simulink model "gm_DUC_1"  (R2024b)
settings: Solver=FixedStepDiscrete  StartTime=0.0  StopTime=50000/fs_duc  FixedStep=1.62760416666667e-07  RelTol=1e-3
undefined symbols (not defined in the file or in its folder): compFilt, hbFilt, lowpassFilt
libraries: simulink x4, dsphdlfiltering2 x3, dsphdlsigops2 x2, hdlmdlgenlib x1, dspsigops x1
settings Model: Creator=31651  LastModifiedBy=31651
settings OptimizationCC: BlockReduction=off  ConditionallyExecuteInputs=off
settings DebuggingCC: SignalRangeChecking=warning  InheritedTsInSrcMsg=none  SingleTaskRateTransMsg=error  ParamPrecisionLossAbsoluteDiffThreshold=0.0001  ParamPrecisionLossRelativeDiffThreshold=0.0001
settings RTWCC: GPUComputeCapability=3.5

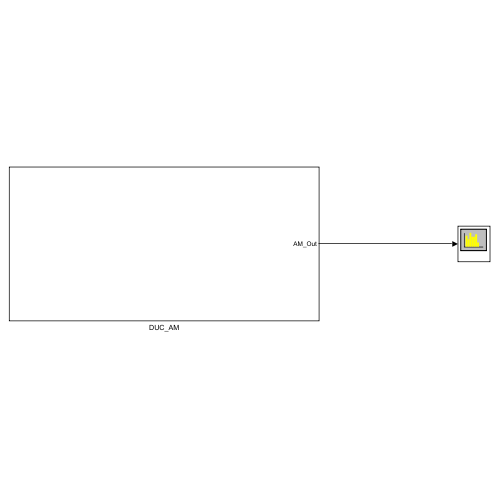
[thumbnail: Simulink's stored preview of the top-level diagram]
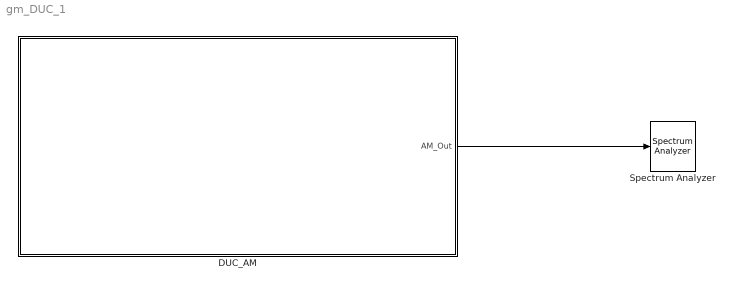
== system gm_DUC_1 ==
  DUC_AM : Subsystem
  Spectrum Analyzer : SpectrumAnalyzer  WindowPosition=[229.000000,148.000000,800.000000,500.000000,]  Visible=on  ScopeFrameLocation=window  SpectrumType=RMS  Method=Welch  WindowInvariantSamplesPerUpdate=on  Span=6144000  StartFrequency=-3072000  StopFrequency=3072000  SpectrumUnits=Vrms  YLimits=[-17.4955218,157.46114017]  SelectedToolstripTab=spectrumAnalyzerToolstrip.estimationTab
  wires:
  DUC_AM/1(AM_Out) -> Spectrum Analyzer/1

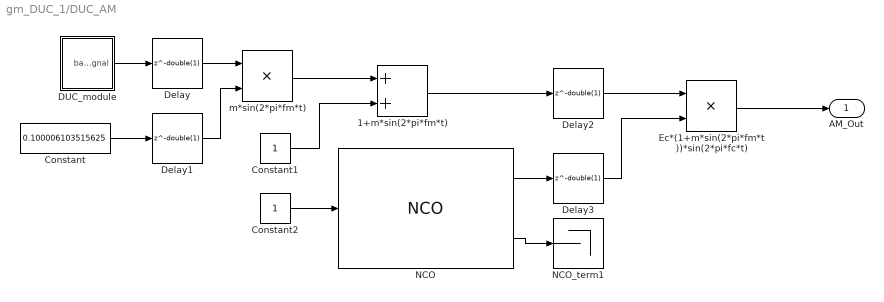
== system gm_DUC_1/DUC_AM ==
  1+m*sin(2*pi*fm*t) : Sum  OutDataTypeStr=fixdt(1, 32, 17)  AccumDataTypeStr=fixdt(1, 32, 17)  SampleTime=1.62760416666667e-07
  Constant : Constant  Value=0.100006103515625  OutDataTypeStr=fixdt(1, 16, 15)  SampleTime=1.62760416666667e-07
  Constant1 : Constant  OutDataTypeStr=int8  SampleTime=1.62760416666667e-07
  Constant2 : Constant  OutDataTypeStr=boolean  SampleTime=1.62760416666667e-07
  DUC_module : Subsystem
  Delay{,1..3} (4 alike) : Delay  DelayLength=double(1)  InitialCondition=0  SampleTime=1.62760416666667e-07
  Ec*(1+m*sin(2*pi*fm*t))*sin(2*pi*fc*t) : Product  Inputs=**  OutDataTypeStr=fixdt(1, 64, 34)  SampleTime=1.62760416666667e-07
  NCO : dsphdlsigops2/NCO  PhaseIncrementSource=Property  PhaseIncrement=phInc  PhaseOffsetSource=Property  PhaseOffset=0  DitherSource=Property  NumDitherBits=ditherBits  SamplesPerFrame=1  LUTCompress=off  ResetAction=off  Waveform=Sine  PhasePort=off  SimulateUsing=Code generation  AccumulatorWL=Nnco  PhaseQuantization=on  NumQuantizerAccumulatorBits=Q  OutputDataType=Binary point scaling  OutputWL=32  OutputFL=17
      settings: LibrarySourceBlock=dsphdlsrcs2/NCO
  NCO_term1 : Terminator
  m*sin(2*pi*fm*t) : Product  Inputs=**  OutDataTypeStr=fixdt(1, 32, 17)  SampleTime=1.62760416666667e-07
  AM_Out : Outport  SampleTime=1.62760416666667e-07
  wires:
  Constant1/1 -> 1+m*sin(2*pi*fm*t)/2
  Constant2/1 -> NCO/1
  DUC_module/1(baseSignal) -> Delay/1
  Constant/1 -> Delay1/1
  Delay/1 -> m*sin(2*pi*fm*t)/1
  Delay1/1 -> m*sin(2*pi*fm*t)/2
  m*sin(2*pi*fm*t)/1 -> 1+m*sin(2*pi*fm*t)/1
  1+m*sin(2*pi*fm*t)/1 -> Delay2/1
  NCO/1 -> Delay3/1
  NCO/2 -> NCO_term1/1
  Delay2/1 -> Ec*(1+m*sin(2*pi*fm*t))*sin(2*pi*fc*t)/1
  Delay3/1 -> Ec*(1+m*sin(2*pi*fm*t))*sin(2*pi*fc*t)/2
  Ec*(1+m*sin(2*pi*fm*t))*sin(2*pi*fc*t)/1 -> AM_Out/1

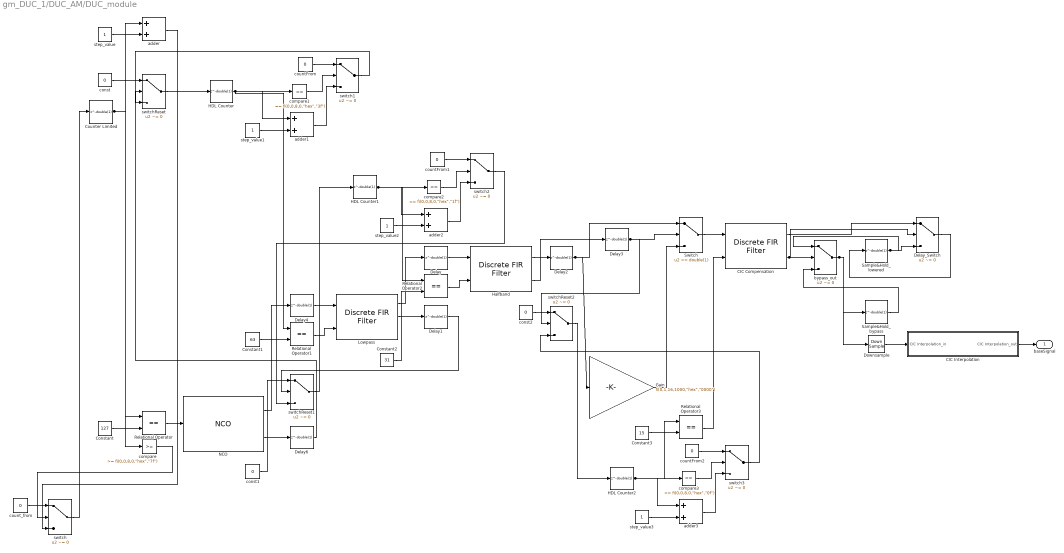
== system gm_DUC_1/DUC_AM/DUC_module ==
  CIC Compensation : dsphdlfiltering2/Discrete FIR Filter  NumeratorSource=Property  Numerator=compFilt.Numerator  NumeratorPrototype=[]  FilterStructure=Direct form systolic  SerializationOption=Minimum number of cycles between valid input samples  NumCycles=2  NumberOfMultipliers=2  SimulateUsing=Code generation  roundingMode=Floor  overflowMode=off  CoefficientsDataTypeStr=Inherit: Same word length as input  OutputDataTypeStr=fixdt(1,16,14)  ResetInputPort=off  HDLGlobalReset=off  CoeffMultiplier=Multiplier  UseMultForPow2Coeff=on
  CIC Interpolation : Subsystem
  Constant : Constant  Value=127  OutDataTypeStr=uint8  SampleTime=1.62760416666667e-07
  Constant1 : Constant  Value=63  OutDataTypeStr=uint8  SampleTime=1.62760416666667e-07
  Constant2 : Constant  Value=31  OutDataTypeStr=uint8  SampleTime=1.62760416666667e-07
  Constant3 : Constant  Value=15  OutDataTypeStr=uint8  SampleTime=1.62760416666667e-07
  Counter Limited : Delay  DelayLength=double(1)  InitialCondition=0  SampleTime=1.62760416666667e-07
  Delay{,1..4,6} (6 alike) : Delay  DelayLength=double(1)  InitialCondition=0  SampleTime=1.62760416666667e-07
  Delay_Switch : Switch  Criteria=u2 ~= 0  Threshold=double(0)  OutDataTypeStr=fixdt(1, 16, 14)  SampleTime=1.62760416666667e-07  SaturateOnIntegerOverflow=off  InputSameDT=off
  Downsample : DownSample  N=double(16)  phase=double(0)  RateOptions=Allow multirate processing  AllowArbitraryFixedInput=on
  Gain : Gain  Gain="fi(0,1,16,1000,\"hex\",\"0000\")"  ParamDataTypeStr=fixdt(1, 16, 1000)  OutDataTypeStr=fixdt(1, 32, 1014)  SampleTime=1.62760416666667e-07
  HDL Counter : Delay  DelayLength=double(1)  InitialCondition=0  SampleTime=1.62760416666667e-07
  HDL Counter1 : Delay  DelayLength=double(1)  InitialCondition=0  SampleTime=1.62760416666667e-07
  HDL Counter2 : Delay  DelayLength=double(1)  InitialCondition=0  SampleTime=1.62760416666667e-07
  Halfband : dsphdlfiltering2/Discrete FIR Filter  NumeratorSource=Property  Numerator=hbFilt.Numerator  NumeratorPrototype=[]  FilterStructure=Direct form systolic  SerializationOption=Minimum number of cycles between valid input samples  NumCycles=2  NumberOfMultipliers=2  SimulateUsing=Code generation  roundingMode=Floor  overflowMode=off  CoefficientsDataTypeStr=Inherit: Same word length as input  OutputDataTypeStr=fixdt(1,16,14)  ResetInputPort=off  HDLGlobalReset=off  CoeffMultiplier=Multiplier  UseMultForPow2Coeff=on
  Lowpass : dsphdlfiltering2/Discrete FIR Filter  NumeratorSource=Property  Numerator=lowpassFilt.Numerator  NumeratorPrototype=[]  FilterStructure=Partly serial systolic  SerializationOption=Maximum number of multipliers  NumCycles=2  NumberOfMultipliers=3  SimulateUsing=Code generation  roundingMode=Floor  overflowMode=off  CoefficientsDataTypeStr=Inherit: Same word length as input  OutputDataTypeStr=fixdt(1,16,14)  ResetInputPort=off  HDLGlobalReset=off  CoeffMultiplier=Multiplier  UseMultForPow2Coeff=on
  NCO : dsphdlsigops2/NCO  PhaseIncrementSource=Property  PhaseIncrement=phInc_b0  PhaseOffsetSource=Property  PhaseOffset=0  DitherSource=Property  NumDitherBits=ditherBits_base  SamplesPerFrame=1  LUTCompress=off  ResetAction=off  Waveform=Sine  PhasePort=off  SimulateUsing=Code generation  AccumulatorWL=Nnco_base  PhaseQuantization=on  NumQuantizerAccumulatorBits=Q_base  OutputDataType=Binary point scaling  OutputWL=16  OutputFL=14
      settings: LibrarySourceBlock=dsphdlsrcs2/NCO
  Relational Operator{,1..3} (4 alike) : RelationalOperator  Operator===  OutDataTypeStr=boolean  SampleTime=1.62760416666667e-07  InputSameDT=off
  Sample&Hold_bypass : Delay  DelayLength=double(1)  InitialCondition=0  SampleTime=1.62760416666667e-07
  Sample&Hold_lowered : Delay  DelayLength=double(1)  InitialCondition=0  SampleTime=1.62760416666667e-07
  Switch : Switch  Threshold=double(1)  OutDataTypeStr=fixdt(1, 16, 14)  SampleTime=1.62760416666667e-07  SaturateOnIntegerOverflow=off  InputSameDT=off
  adder{,1..3} (4 alike) : Sum  OutDataTypeStr=uint8  AccumDataTypeStr=uint8  SampleTime=1.62760416666667e-07
  bypass_out : Switch  Criteria=u2 ~= 0  Threshold=double(0)  OutDataTypeStr=fixdt(1, 16, 14)  SampleTime=1.62760416666667e-07  SaturateOnIntegerOverflow=off  InputSameDT=off
  compare : simulink/Logic and Bit Operations/Compare To Constant  relop=>=  const="fi(0,0,8,0,\"hex\",\"7f\")"  OutDataTypeStr=boolean
  compare1 : simulink/Logic and Bit Operations/Compare To Constant  relop===  const="fi(0,0,8,0,\"hex\",\"3f\")"  OutDataTypeStr=boolean
  compare2 : simulink/Logic and Bit Operations/Compare To Constant  relop===  const="fi(0,0,8,0,\"hex\",\"1f\")"  OutDataTypeStr=boolean
  compare3 : simulink/Logic and Bit Operations/Compare To Constant  relop===  const="fi(0,0,8,0,\"hex\",\"0f\")"  OutDataTypeStr=boolean
  const : Constant  Value=0  VectorParams1D=off  OutDataTypeStr=uint8  SampleTime=1.62760416666667e-07
  const1 : Constant  Value=0  VectorParams1D=off  OutDataTypeStr=uint8  SampleTime=1.62760416666667e-07
  const2 : Constant  Value=0  VectorParams1D=off  OutDataTypeStr=uint8  SampleTime=1.62760416666667e-07
  countFrom : Constant  Value=0  VectorParams1D=off  OutDataTypeStr=uint8  SampleTime=1.62760416666667e-07
  countFrom1 : Constant  Value=0  VectorParams1D=off  OutDataTypeStr=uint8  SampleTime=1.62760416666667e-07
  countFrom2 : Constant  Value=0  VectorParams1D=off  OutDataTypeStr=uint8  SampleTime=1.62760416666667e-07
  count_from : Constant  Value=0  VectorParams1D=off  OutDataTypeStr=uint8  SampleTime=1.62760416666667e-07
  step_value{,1..3} (4 alike) : Constant  VectorParams1D=off  OutDataTypeStr=uint8  SampleTime=1.62760416666667e-07
  switch{,1..3} (4 alike) : Switch  Criteria=u2 ~= 0  Threshold=double(0)  OutDataTypeStr=uint8  SampleTime=1.62760416666667e-07  SaturateOnIntegerOverflow=off  InputSameDT=off
  switchReset : Switch  Criteria=u2 ~= 0  Threshold=double(0)  OutDataTypeStr=uint8  SampleTime=1.62760416666667e-07  SaturateOnIntegerOverflow=off  InputSameDT=off
  switchReset1 : Switch  Criteria=u2 ~= 0  Threshold=double(0)  OutDataTypeStr=uint8  SampleTime=1.62760416666667e-07  SaturateOnIntegerOverflow=off  InputSameDT=off
  switchReset2 : Switch  Criteria=u2 ~= 0  Threshold=double(0)  OutDataTypeStr=uint8  SampleTime=1.62760416666667e-07  SaturateOnIntegerOverflow=off  InputSameDT=off
  baseSignal : Outport  SampleTime=1.62760416666667e-07
  wires:
  CIC Interpolation/1(CIC Interpolation_out) -> baseSignal/1
  const/1 -> switchReset/1
  countFrom2/1 -> switch3/1
  count_from/1 -> switch/1
  CIC Compensation/1 -> Delay_Switch/1
  switch/1 -> Counter Limited/1
  step_value/1 -> adder/2
  Counter Limited/1 -> compare/1, adder/1, Relational Operator/1
  Constant/1 -> Relational Operator/2
  Sample&Hold_bypass/1 -> bypass_out/3
  Delay6/1 -> switchReset/2
  switchReset/1 -> HDL Counter/1
  adder/1 -> switch/3
  step_value1/1 -> adder1/2
  Relational Operator/1 -> NCO/1
  compare/1 -> switch/2
  Relational Operator3/1 -> CIC Compensation/2
  switchReset1/1 -> HDL Counter1/1
  HDL Counter/1 -> adder1/1, compare1/1, Relational Operator1/1
  Constant1/1 -> Relational Operator1/2
  step_value2/1 -> adder2/2
  NCO/1 -> Delay4/1
  const2/1 -> switchReset2/1
  NCO/2 -> Delay6/1
  Downsample/1 -> CIC Interpolation/1(CIC Interpolation_in)
  const1/1 -> switchReset1/1
  countFrom/1 -> switch1/1
  compare1/1 -> switch1/2
  adder1/1 -> switch1/3
  Delay4/1 -> Lowpass/1
  Relational Operator1/1 -> Lowpass/2
  switch1/1 -> switchReset/3
  HDL Counter1/1 -> adder2/1, compare2/1, Relational Operator2/1
  Delay1/1 -> switchReset1/2
  Lowpass/2 -> Delay1/1
  Lowpass/1 -> Delay/1
  Constant2/1 -> Relational Operator2/2
  Switch/1 -> CIC Compensation/1
  countFrom1/1 -> switch2/1
  compare2/1 -> switch2/2
  adder2/1 -> switch2/3
  Relational Operator2/1 -> Halfband/2
  Delay/1 -> Halfband/1
  switch2/1 -> switchReset1/3
  Halfband/1 -> Delay2/1
  Halfband/2 -> Delay3/1
  Delay2/1 -> Switch/1, Gain/1
  switchReset2/1 -> HDL Counter2/1
  CIC Compensation/2 -> Delay_Switch/2, bypass_out/2
  Gain/1 -> Switch/3
  Delay3/1 -> switchReset2/2, Switch/2
  Constant3/1 -> Relational Operator3/2
  Delay_Switch/1 -> Sample&Hold_lowered/1
  HDL Counter2/1 -> adder3/1, compare3/1, Relational Operator3/1
  step_value3/1 -> adder3/2
  compare3/1 -> switch3/2
  adder3/1 -> switch3/3
  switch3/1 -> switchReset2/3
  bypass_out/1 -> Downsample/1, Sample&Hold_bypass/1
  Sample&Hold_lowered/1 -> bypass_out/1, Delay_Switch/3

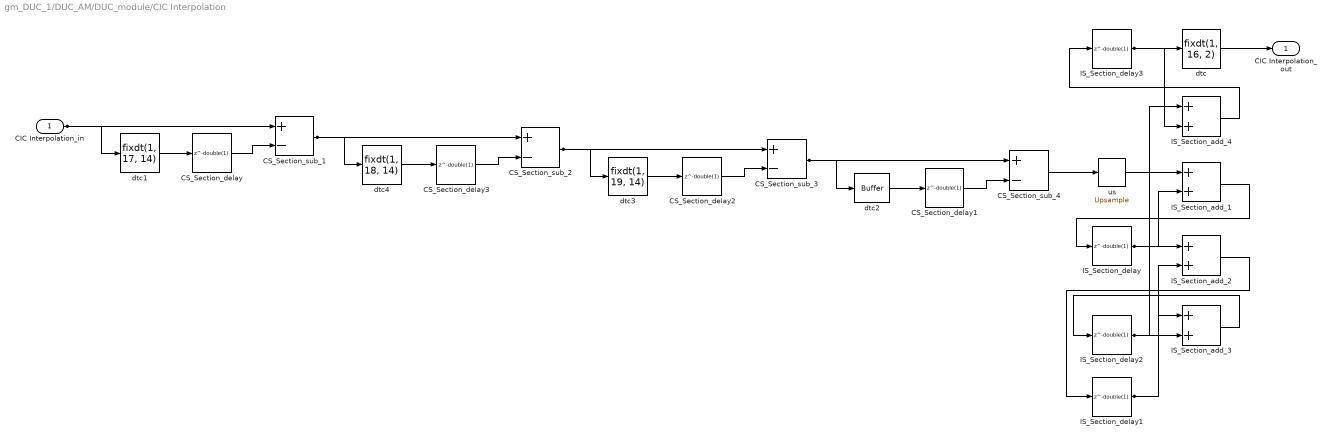
== system gm_DUC_1/DUC_AM/DUC_module/CIC Interpolation ==
  CIC Interpolation_in : Inport  OutDataTypeStr=fixdt(1, 16, 14)  SampleTime=2.60416666666667e-06
  CS_Section_delay{,1..3} (4 alike) : Delay  DelayLength=double(1)  InitialCondition=0  SampleTime=2.60416666666667e-06
  CS_Section_sub_1 : Sum  Inputs=+-  OutDataTypeStr=fixdt(1, 17, 14)  SampleTime=2.60416666666667e-06
  CS_Section_sub_2 : Sum  Inputs=+-  OutDataTypeStr=fixdt(1, 18, 14)  SampleTime=2.60416666666667e-06
  CS_Section_sub_3 : Sum  Inputs=+-  OutDataTypeStr=fixdt(1, 19, 14)  SampleTime=2.60416666666667e-06
  CS_Section_sub_4 : Sum  Inputs=+-  OutDataTypeStr=fixdt(1, 19, 14)  SampleTime=2.60416666666667e-06
  IS_Section_add_1 : Sum  OutDataTypeStr=fixdt(1, 19, 14)  SampleTime=1.62760416666667e-07
  IS_Section_add_2 : Sum  OutDataTypeStr=fixdt(1, 22, 14)  SampleTime=1.62760416666667e-07
  IS_Section_add_3 : Sum  OutDataTypeStr=fixdt(1, 25, 14)  SampleTime=1.62760416666667e-07
  IS_Section_add_4 : Sum  OutDataTypeStr=fixdt(1, 28, 14)  SampleTime=1.62760416666667e-07
  IS_Section_delay{,1..3} (4 alike) : Delay  DelayLength=double(1)  InitialCondition=0  SampleTime=1.62760416666667e-07
  dtc : DataTypeConversion  OutDataTypeStr=fixdt(1, 16, 2)  SampleTime=1.62760416666667e-07  SaturateOnIntegerOverflow=off  RndMeth=Floor
  dtc1 : DataTypeConversion  OutDataTypeStr=fixdt(1, 17, 14)  SampleTime=2.60416666666667e-06  SaturateOnIntegerOverflow=off  RndMeth=Floor
  dtc2 : hdlmdlgenlib/Buffer
  dtc3 : DataTypeConversion  OutDataTypeStr=fixdt(1, 19, 14)  SampleTime=2.60416666666667e-06  SaturateOnIntegerOverflow=off  RndMeth=Floor
  dtc4 : DataTypeConversion  OutDataTypeStr=fixdt(1, 18, 14)  SampleTime=2.60416666666667e-06  SaturateOnIntegerOverflow=off  RndMeth=Floor
  us : dspsigops/Upsample  FactorSource=Dialog parameter  N=double(16)  Nmax=16  phase=double(0)  RateOptions=Allow multirate processing  ic=0  mode=Unused parameter value
  CIC Interpolation_out : Outport  OutDataTypeStr=fixdt(1, 16, 2)  SampleTime=1.62760416666667e-07
  wires:
  dtc1/1 -> CS_Section_delay/1
  dtc2/1 -> CS_Section_delay1/1
  CIC Interpolation_in/1 -> dtc1/1, CS_Section_sub_1/1
  CS_Section_delay/1 -> CS_Section_sub_1/2
  CS_Section_sub_2/1 -> dtc3/1, CS_Section_sub_3/1
  CS_Section_delay3/1 -> CS_Section_sub_2/2
  dtc/1 -> CIC Interpolation_out/1
  CS_Section_sub_1/1 -> CS_Section_sub_2/1, dtc4/1
  dtc4/1 -> CS_Section_delay3/1
  dtc3/1 -> CS_Section_delay2/1
  IS_Section_delay2/1 -> IS_Section_add_4/1, IS_Section_add_3/2
  CS_Section_delay2/1 -> CS_Section_sub_3/2
  CS_Section_sub_3/1 -> CS_Section_sub_4/1, dtc2/1
  CS_Section_delay1/1 -> CS_Section_sub_4/2
  CS_Section_sub_4/1 -> us/1
  IS_Section_delay3/1 -> IS_Section_add_4/2, dtc/1
  us/1 -> IS_Section_add_1/1
  IS_Section_delay/1 -> IS_Section_add_2/1, IS_Section_add_1/2
  IS_Section_delay1/1 -> IS_Section_add_2/2, IS_Section_add_3/1
  IS_Section_add_4/1 -> IS_Section_delay3/1
  IS_Section_add_1/1 -> IS_Section_delay/1
  IS_Section_add_2/1 -> IS_Section_delay1/1
  IS_Section_add_3/1 -> IS_Section_delay2/1
